simulink model "tes_3phaseSIM"  (R2016a)
settings: Solver=VariableStepAuto  StartTime=0.0  StopTime=10.0  RelTol=1e-3
settings Model: Creator=krishna  LastModifiedBy=krishna

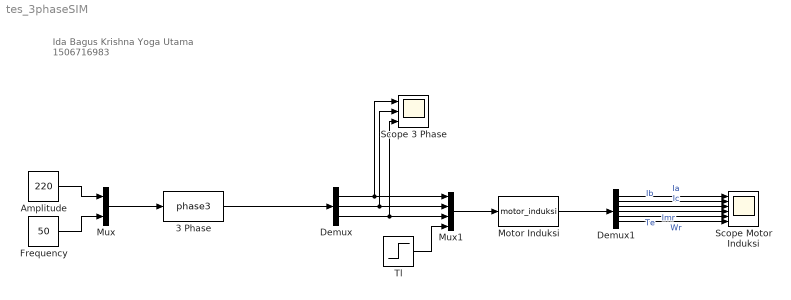
== system tes_3phaseSIM ==
  note: Ida Bagus Krishna Yoga Utama
      | 1506716983
  3 Phase : S-Function  FunctionName=phase3  SFunctionDeploymentMode=off  EnableBusSupport=off
  Amplitude : Constant  Value=220
  Demux : Demux  Outputs=3
  Demux1 : Demux  Outputs=6
  Frequency : Constant  Value=50
  Motor Induksi : S-Function  FunctionName=motor_induksi  SFunctionDeploymentMode=off  EnableBusSupport=off
  Mux : Mux  Inputs=2
  Mux1 : Mux
  Scope 3 Phase : Scope  NumInputPorts=3
  Scope Motor Induksi : Scope  NumInputPorts=6
  Tl : Step  Time=10  SampleTime=0
  wires:
  Amplitude/1 -> Mux/1
  Frequency/1 -> Mux/2
  Mux/1 -> 3 Phase/1
  3 Phase/1 -> Demux/1
  Demux/1 -> Scope 3 Phase/1, Mux1/1
  Demux/2 -> Scope 3 Phase/2, Mux1/2
  Demux/3 -> Scope 3 Phase/3, Mux1/3
  Mux1/1 -> Motor Induksi/1
  Motor Induksi/1 -> Demux1/1
  Demux1/1 -> Scope Motor Induksi/1  "Ia"
  Demux1/2 -> Scope Motor Induksi/2  "Ib"
  Demux1/3 -> Scope Motor Induksi/3  "Ic"
  Demux1/4 -> Scope Motor Induksi/4  "Imr"
  Demux1/5 -> Scope Motor Induksi/5  "Te"
  Demux1/6 -> Scope Motor Induksi/6  "Wr"
  Tl/1 -> Mux1/4
